simulink model "Position_control"  (R2022a)
settings: Solver=FixedStepAuto  StartTime=0.0  StopTime=inf  RelTol=1e-3  EnableMultiTasking=on
undefined symbols (not defined in the file): kd2, kp2
libraries: arduinolib x3, arduinosensorlib x1, simulink_extras x1
settings Model: ExtModeTrigDuration=2  Creator=LabPC  LastModifiedBy=LabPC
settings OptimizationCC: EnhancedBackFolding=on  PassReuseOutputArgsAs=Individual arguments  ZeroExternalMemoryAtStartup=off  ZeroInternalMemoryAtStartup=off  MaxStackSize=64  OptimizeBlockOrder=speed  DifferentSizesBufferReuse=on  OptimizationCustomize=off  EfficientTunableParamExpr=on
settings DebuggingCC: ParameterTunabilityLossMsg=error
settings HardwareCC: ProdBitPerInt=16  ProdBitPerPointer=16  ProdBitPerSizeT=16  ProdBitPerPtrDiffT=16  ProdLargestAtomicFloat=None  ProdWordSize=8  ProdHWDeviceType=Atmel->AVR
settings SFSimCC: MATLABDynamicMemAlloc=off
settings RTWCC: SystemTargetFile=ert.tlc  HardwareBoard=Arduino Mega 2560  TemplateMakefile=ert_default_tmf  Toolchain=Arduino AVR  BuildConfiguration=Faster Runs
settings CodeAppCC: ForceParamTrailComments=on  IgnoreCustomStorageClasses=off  OperatorAnnotations=on  SimulinkDataObjDesc=on  SFDataObjDesc=on  InsertBlockDesc=on
settings ERTTargetCC: SupportContinuousTime=on  SupportVariableSizeSignals=on  ExtModeTransport=3  ExtModeStaticAlloc=on  ExtModeStaticAllocSize=2048  ExtModeMexFile=ext_xcp  ExtModeIntrfLevel=Level2 - Open

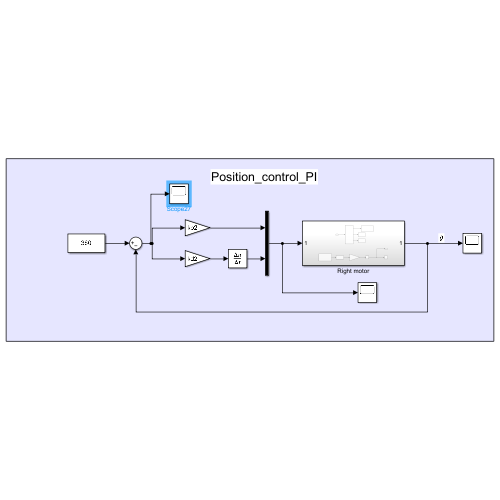
[thumbnail: Simulink's stored preview of the top-level diagram]
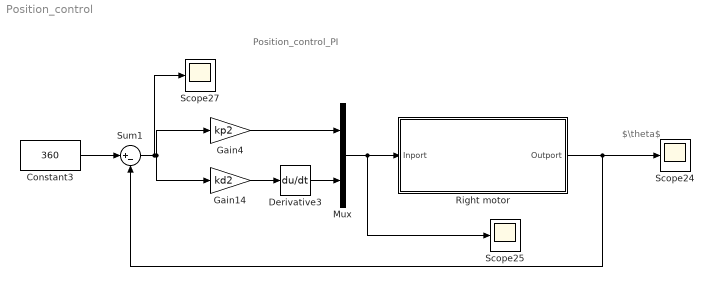
== system Position_control ==
  note: Position_control_PI
  note: $\theta$
  Constant3 : Constant  Value=360
  Derivative3 : Derivative
  Gain14 : Gain  Gain=kd2
  Gain4 : Gain  Gain=kp2
  Mux : Mux  Inputs=2
  Right motor : Subsystem
  Scope24 : Scope
  Scope25 : Scope
  Scope27 : Scope
  Sum1 : Sum  Inputs=|+-
  wires:
  Gain4/1 -> Mux/1
  Derivative3/1 -> Mux/2
  Gain14/1 -> Derivative3/1
  Mux/1 -> Right motor/1(Inport), Scope25/1
  Constant3/1 -> Sum1/1
  Right motor/1(Outport) -> Sum1/2, Scope24/1
  Sum1/1 -> Scope27/1, Gain4/1, Gain14/1

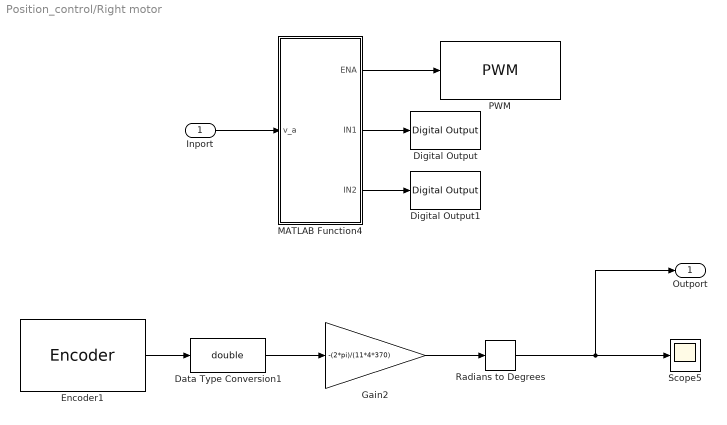
== system Position_control/Right motor ==
  Inport : Inport
  Data Type Conversion1 : DataTypeConversion  OutDataTypeStr=double  SaturateOnIntegerOverflow=off  RndMeth=Floor
  Digital Output : arduinolib/Digital Output  pinNumber=5  Direction=output  blockPlatform=arduino
  Digital Output1 : arduinolib/Digital Output  pinNumber=7  Direction=output  blockPlatform=arduino
  Encoder1 : arduinosensorlib/Encoder  InputA=2  InputB=3  Mode=No reset  SampleTime=-1
      settings: SourceProductBaseCode=ARDUINO
  Gain2 : Gain  Gain=-(2*pi)/(11*4*370)
  MATLAB Function4 : MATLAB Function  TreatAsAtomicUnit=on
  PWM : arduinolib/PWM  pinNumber=4  frequencyType=Default  desiredFrequency=490.2  achievableFrequency=490.2
  Radians to Degrees : simulink_extras/Transformations/Radians to Degrees
  Scope5 : Scope
  Outport : Outport
  wires:
  Data Type Conversion1/1 -> Gain2/1
  Radians to Degrees/1 -> Scope5/1, Outport/1
  MATLAB Function4/3(IN2) -> Digital Output1/1
  MATLAB Function4/2(IN1) -> Digital Output/1
  Gain2/1 -> Radians to Degrees/1
  Encoder1/1 -> Data Type Conversion1/1
  Inport/1 -> MATLAB Function4/1(v_a)
  MATLAB Function4/1(ENA) -> PWM/1

== matlab function Position_control/Right motor/MATLAB Function4 ==
  data: v_a input; ENA output; IN1 output; IN2 output
function [ENA,IN1,IN2] = fcn(v_a)

vmax = 10;
pwm_cal = v_a*254/vmax;

if pwm_cal > 0
    ENA = pwm_cal;
    IN1 = 1;
    IN2 = 0;
elseif pwm_cal < 0
    ENA = abs(pwm_cal);
    IN1 = 0;
    IN2 = 1;
else
    ENA = 0;
    IN1 = 0;
    IN2 = 0;
   
end
